simulink library "TorqueChecker"  (R2016b)
settings: Solver=VariableStepAuto  StartTime=0.0  StopTime=10.0  RelTol=1e-3
undefined symbols (not defined in the file): maxTorque
settings Model: Creator=Marc  LastModifiedBy=march

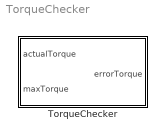
== system TorqueChecker ==
  TorqueChecker : Subsystem

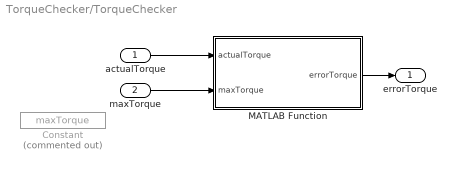
== system TorqueChecker/TorqueChecker ==
  actualTorque : Inport
  maxTorque : Inport  Port=2
  Constant : Constant  Commented=on  Value=maxTorque  VectorParams1D=off  SampleTime=-1
  MATLAB Function : MATLAB Function  TreatAsAtomicUnit=on
  errorTorque : Outport
  wires:
  maxTorque/1 -> MATLAB Function/2(maxTorque)
  MATLAB Function/1(errorTorque) -> errorTorque/1
  actualTorque/1 -> MATLAB Function/1(actualTorque)

== matlab function TorqueChecker/MATLAB Function ==
  data: actualTorque input; errorTorque output; maxTorque input
function errorTorque = fcn(actualTorque, maxTorque)
%MAX TORQUE CHECKER
if abs(actualTorque) >= maxTorque
    errorTorque =1;
else
    errorTorque =0;
end
